simulink model "CounterModel"  (R2024b)
settings: Solver=FixedStepDiscrete  StartTime=0.0  StopTime=48  FixedStep=1  RelTol=1e-3  SampleTimeConstraint=STIndependent  EnableMultiTasking=on
PostLoadFcn:
  | INC = uint8(1);
  | LIMIT = uint8(16);
  | RESET = uint8(0);
  | K = int32(2);
  | coder.example.configure(bdroot, 'ERT');
Description:
  | A simple counter model for code generation and code building examples.
settings Model: ParamWorkspaceSource=ReferencedWorkspace  Creator=The MathWorks, Inc.  LastModifiedBy=The MathWorks, Inc.
settings SolverCC: AlgebraicLoopSolver=TrustRegion
settings DataIOCC: SaveFormat=StructureWithTime  SaveOutput=off  SaveTime=off  ReturnWorkspaceOutputs=off  SignalLoggingName=sigsOut
settings OptimizationCC: DefaultParameterBehavior=Inlined  UseDivisionForNetSlopeComputation=on  InlineInvariantSignals=on  EnhancedBackFolding=on  BooleansAsBitfields=on  PassReuseOutputArgsAs=Individual arguments  ExpressionDepthLimit=2147483647  StateBitsets=on  DataBitsets=on  ZeroExternalMemoryAtStartup=off  ZeroInternalMemoryAtStartup=off  NoFixptDivByZeroProtection=on  EfficientFloat2IntCast=on  BufferReusableBoundary=off  OptimizeBlockOrder=speed  DifferentSizesBufferReuse=on  EfficientTunableParamExpr=on
settings DebuggingCC: MergeDetectMultiDrivingBlocksExec=none  CheckExecutionContextPreStartOutputMsg=on  IntegerOverflowMsg=none  ParameterTunabilityLossMsg=error  FcnCallInpInsideContextMsg=warning  UnconnectedInputMsg=warning  UnconnectedOutputMsg=warning  UnconnectedLineMsg=warning  AllowSymbolicDim=off  StateNameClashWarn=warning  SubsystemReferenceDiagnosticForUnitTest=warning  StrictBusMsg=ErrorOnBusTreatedAsVector  SFUnexpectedBacktrackingDiag=warning  SFNoUnconditionalDefaultTransitionDiag=warning  SFExecutionAtInitializationDiag=none  IntegerSaturationMsg=none  ArithmeticOperatorsInVariantConditions=warning
settings HardwareCC: ProdLargestAtomicFloat=None  ProdLongLongMode=on  ProdHWDeviceType=Specified  TargetHWDeviceType=Generic->32-bit Embedded Processor
settings ModelReferenceCC: UpdateModelReferenceTargets=IfOutOfDate  EnableRefExpFcnMdlSchedulingChecks=on  PropagateSignalLabelsOutOfModel=off
settings SFSimCC: SimUseLocalCustomCode=off  MATLABDynamicMemAlloc=off
settings RTWCC: Description=Embedded Coder  SystemTargetFile=ert.tlc  TLCOptions=-p0 -aWarnNonSaturatedBlocks=0  TemplateMakefile=ert_default_tmf  GenerateReport=on  RTWVerbose=off  RTWUseLocalCustomCode=off  IncludeHyperlinkInReport=on  LaunchReport=on  GenerateTraceInfo=on  GenerateTraceReport=on  GenerateTraceReportSl=on  GenerateTraceReportSf=on  GenerateTraceReportEml=on  GenerateCodeMetricsReport=on  GPUComputeCapability=3.5  DLArmComputeVersion=19.05
settings CodeAppCC: ForceParamTrailComments=on  IgnoreCustomStorageClasses=off  OperatorAnnotations=on  SimulinkDataObjDesc=on  SFDataObjDesc=on  CustomSymbolStrGlobalVar=rt$N$M  CustomSymbolStrType=$N$M  CustomSymbolStrFcn=$N$M$F  CustomSymbolStrMacro=$N$M  InsertBlockDesc=on
settings ERTTargetCC: UtilityFuncGeneration=Shared location  GenerateSampleERTMain=on  IncludeMdlTerminateFcn=off  CombineSignalStateStructs=on  SupportNonFinite=off  SupportComplex=off  ERTCustomFileTemplate=example_file_process.tlc  ERTFilePackagingFormat=CompactWithDataFile
settings ConfigComp: CovMetricSettings=d  CovSaveCumulativeToWorkspaceVar=on  CovSaveSingleToWorkspaceVar=on  CovExternalEMLEnable=off

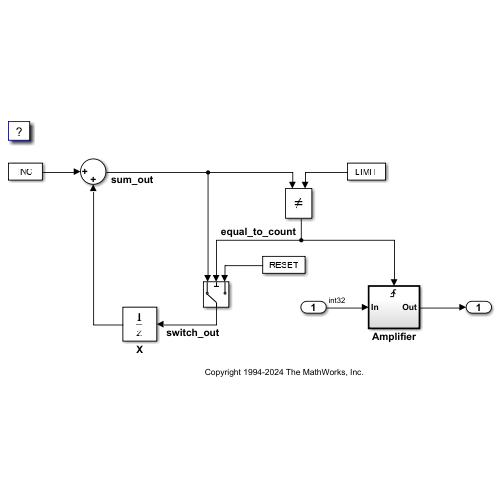
[thumbnail: Simulink's stored preview of the top-level diagram]
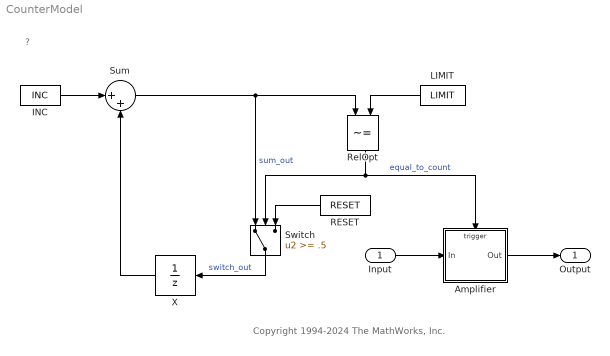
== system CounterModel ==
  note: ?
  note: Copyright 1994-2024 The MathWorks, Inc.
  Input : Inport  OutDataTypeStr=int32  PortDimensions=1
  Amplifier : Subsystem  TreatAsAtomicUnit=on
  INC : Constant  Value=INC
  LIMIT : Constant  Value=LIMIT
  RESET : Constant  Value=RESET
  RelOpt : RelationalOperator  Operator=~=  OutDataTypeStr=boolean
  Sum : Sum  Inputs=|++  InputSameDT=on  OutDataTypeStr=Inherit: Same as first input
  Switch : Switch  Threshold=.5  SaturateOnIntegerOverflow=off
  X : UnitDelay  SampleTime=-1  StateName=X  HasFrameUpgradeWarning=on
  Output : Outport  VectorParamsAs1DForOutWhenUnconnected=off
  wires:
  INC/1 -> Sum/1
  X/1 -> Sum/2
  Switch/1 -> X/1  "switch_out"
  Sum/1 -> Switch/1, RelOpt/1  "sum_out"
  LIMIT/1 -> RelOpt/2
  Input/1 -> Amplifier/1(In)
  RESET/1 -> Switch/3
  RelOpt/1 -> Switch/2, Amplifier/Trigger  "equal_to_count"
  Amplifier/1(Out) -> Output/1

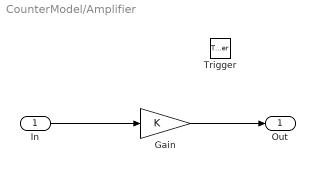
== system CounterModel/Amplifier ==
  In : Inport
  Trigger : TriggerPort  VariantControl=Variant
  Gain : Gain  Gain=K  OutDataTypeStr=Inherit: Same as input  ParamDataTypeStr=Inherit: Same as input
  Out : Outport  InitialOutput=0  VectorParamsAs1DForOutWhenUnconnected=off
  wires:
  In/1 -> Gain/1
  Gain/1 -> Out/1
